simulink model "cruise_control_sim"  (R2017b)
settings: Solver=ode1  StartTime=0.0  StopTime=50  FixedStep=0.1  RelTol=1e-3
values from neighbouring files (symbols this model uses):
  EngineRPM = [1000 1500 2000 2500 3000 3500 4000 4500 5000 5500 6000 6500 ... (13 elements, 1x13)]    [alpha147gta.mat]    (also in cruise_control_external.mat; cruise_control_sim.mat)
  EngineTRQ = [200 220 242 258 260 261 268 285 300 296 290 250 ... (13 elements, 1x13)]    [alpha147gta.mat]    (also in cruise_control_external.mat; cruise_control_sim.mat)
  FinalRatio = 3.733    [alpha147gta.mat]    (also in cruise_control_external.mat; cruise_control_sim.mat)
  GearRatio = [3.5 2.235 1.52 1.156 0.971 0.818]    [alpha147gta.mat]    (also in cruise_control_external.mat; cruise_control_sim.mat)
  Kdrag = 0.4238432    [alpha147gta.mat]    (also in cruise_control_external.mat; cruise_control_sim.mat)
  Ki = 1    [cruise_control.mat]    (also in cruise_control_external.mat = 0.002; cruise_control_sim.mat = 0.002)
  Kp = 1    [cruise_control.mat]    (also in cruise_control_external.mat = 0.4; cruise_control_sim.mat = 0.4)
  Mass = 1360    [alpha147gta.mat]    (also in cruise_control_external.mat; cruise_control_sim.mat)
  WheelRadius = 0.2992    [alpha147gta.mat]    (also in cruise_control_external.mat; cruise_control_sim.mat)
undefined symbols (not defined in the file or in its folder): sigbuilder_block
settings Model: Creator=Rehaan M. Bhimani  LastModifiedBy=Rehaan M. Bhimani

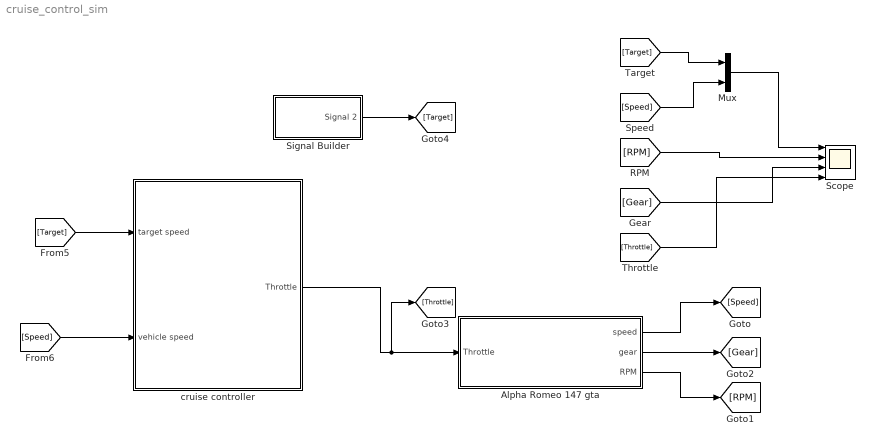
== system cruise_control_sim ==
  Alpha Romeo 147 gta : Subsystem
  Mux : Mux  Inputs=2
  Scope : Scope  NumInputPorts=4
  Signal Builder : Subsystem  Tag=STV Subsys  LoadFcn=sigbuilder_block('load');  StartFcn=sigbuilder_block('start');  StopFcn=sigbuilder_block('stop');  ClipboardFcn=sigbuilder_block('clipboard');  mask(Sigbuilder block){tuvar=[0:10]}
      mask help: Simulink:masks:SigbuilderBlock_MD
      mask init:
      | if ~strcmp(get_param(bdroot(gcbh),'SimulationStatus'),'stopped') tuvar = sigbuilder_block('maskInit'); end
      settings: CopyFcn=sigbuilder_block('copy');  DeleteFcn=sigbuilder_block('delete');  ModelCloseFcn=sigbuilder_block('modelClose');  PreSaveFcn=sigbuilder_block('preSave');  PauseFcn=sigbuilder_block('pause');  ContinueFcn=sigbuilder_block('continue');  NameChangeFcn=sigbuilder_block('namechange');  OpenFcn=sigbuilder_block('open',[404 117.5 550.5 362.5 ]);  CloseFcn=sigbuilder_block('close');
      mask Display: plot(0, 0, 100, 100,[2, 2, 32, 32, 2], [68, 8, 8, 68, 68],[32, 2], [38, 38], [32, 19, 2],[53, 60, 44], [32, 17, 17, 2],[16, 16, 31, 31]);txt = getActiveGroup(gcbh);text(2, 100, txt,'verticalAlignment', 'top');
  "cruise controller " : Subsystem
  wires:
  "cruise controller "/1("Throttle ") -> [Throttle], Alpha Romeo 147 gta/1(Throttle)
  [Target] -> "cruise controller "/1(target speed)
  Alpha Romeo 147 gta/1(speed) -> [Speed]
  Alpha Romeo 147 gta/2(gear) -> [Gear]
  Alpha Romeo 147 gta/3(RPM) -> [RPM]
  [Speed] -> "cruise controller "/2(vehicle speed)
  [Target] -> Mux/1
  [Speed] -> Mux/2
  Mux/1 -> Scope/1
  [RPM] -> Scope/2
  [Gear] -> Scope/3
  [Throttle] -> Scope/4
  Signal Builder/1(Signal 2) -> [Target]

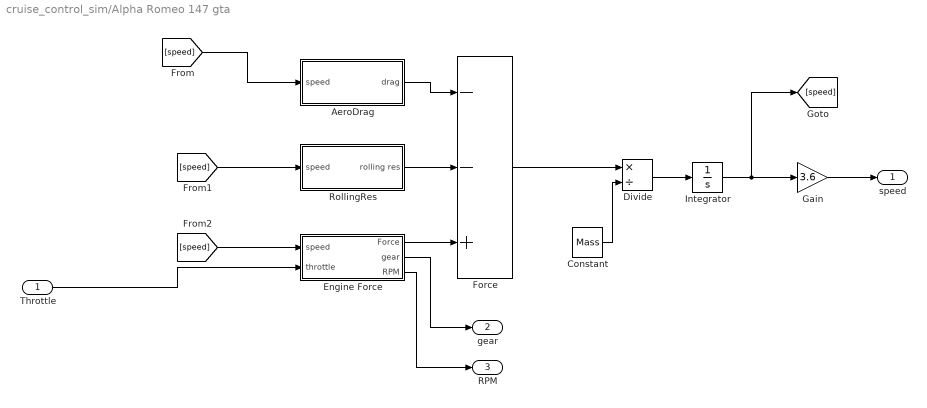
== system cruise_control_sim/Alpha Romeo 147 gta ==
  Throttle : Inport
  AeroDrag : Subsystem
  Constant : Constant  Value=Mass
  Divide : Product  Inputs=*/
  Engine Force : Subsystem
  Force : Sum  Inputs=--+
  Gain : Gain  Gain=3.6
  Integrator : Integrator
  RollingRes : Subsystem
  speed : Outport
  gear : Outport  Port=2
  RPM : Outport  Port=3
  wires:
  Throttle/1 -> Engine Force/2(throttle)
  [speed] -> Engine Force/1(speed)
  Gain/1 -> speed/1
  Force/1 -> Divide/1
  RollingRes/1(rolling res) -> Force/2
  AeroDrag/1(drag) -> Force/1
  [speed] -> RollingRes/1(speed)
  Engine Force/1(Force) -> Force/3
  Divide/1 -> Integrator/1
  Integrator/1 -> [speed], Gain/1
  Constant/1 -> Divide/2
  [speed] -> AeroDrag/1(speed)
  Engine Force/2(gear) -> gear/1
  Engine Force/3(RPM) -> RPM/1

== system cruise_control_sim/Signal Builder ==
  Demux : Demux  Tag=STV Demux  Outputs=1
  FromWs : FromWorkspace  Tag=STV FromWs  VariableName=tuvar  SampleTime=0
      SigBuilderData=|
      | common.afterFinalStr = 'Extrapolate'
      | common.sampleTime = 0
      | dataSet.timeRange = [0 50]
      | dataSet.name = 'Group 1'
      | sbobj.Groups.Name = 'Group 1'
      | sbobj.Groups.Signals.Name = 'Signal 2'
      | sbobj.Groups.Signals.XData = [0 5 5 10 10 20 20 30 30 40 40 50]
      | sbobj.Groups.Signals.YData = [30 30 50 50 80 80 100 100 120 120 140 140]
      | sbobj.Groups.TimeRange = [0 50]
  Signal 2 : Outport  Tag=STV Outport
  wires:
  FromWs/1 -> Demux/1
  Demux/1 -> Signal 2/1

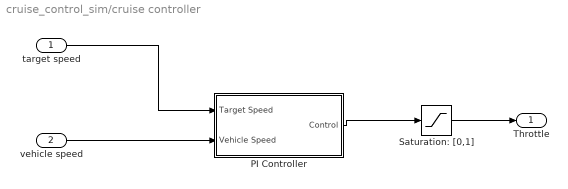
== system cruise_control_sim/cruise controller  ==
  target speed : Inport
  vehicle speed : Inport  Port=2
  PI Controller : Subsystem
  Saturation: [0,1] : Saturate  UpperLimit=1  LowerLimit=0
  "Throttle " : Outport
  wires:
  Saturation: [0,1]/1 -> "Throttle "/1
  target speed/1 -> PI Controller/1(Target Speed)
  vehicle speed/1 -> PI Controller/2(Vehicle Speed)
  PI Controller/1(Control) -> Saturation: [0,1]/1

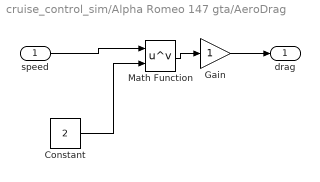
== system cruise_control_sim/Alpha Romeo 147 gta/AeroDrag ==
  speed : Inport
  Constant : Constant  Value=2
  Gain : Gain
  Math Function : Math  Operator=pow  SaturateOnIntegerOverflow=on
  drag : Outport
  wires:
  Gain/1 -> drag/1
  Math Function/1 -> Gain/1
  Constant/1 -> Math Function/2
  speed/1 -> Math Function/1

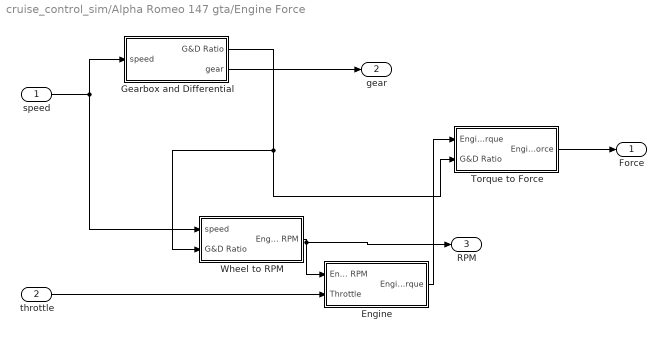
== system cruise_control_sim/Alpha Romeo 147 gta/Engine Force ==
  speed : Inport
  throttle : Inport  Port=2
  Engine : Subsystem
  Gearbox and Differential : Subsystem
  Torque to Force : Subsystem
  Wheel to RPM : Subsystem
  Force : Outport
  gear : Outport  Port=2
  RPM : Outport  Port=3
  wires:
  speed/1 -> Wheel to RPM/1(speed), Gearbox and Differential/1(speed)
  throttle/1 -> Engine/2(Throttle)
  Gearbox and Differential/1(G&D Ratio) -> Torque to Force/2(G&D Ratio), Wheel to RPM/2(G&D Ratio)
  Wheel to RPM/1(Engine RPM) -> RPM/1, Engine/1("Engine RPM ")
  Engine/1(Engine Torque) -> Torque to Force/1(Engine Torque)
  Torque to Force/1(Engine Force) -> Force/1
  Gearbox and Differential/2(gear) -> gear/1

== system cruise_control_sim/Alpha Romeo 147 gta/RollingRes ==
  speed : Inport
  Gain : Gain  Gain=30 * Kdrag
  rolling res : Outport
  wires:
  speed/1 -> Gain/1
  Gain/1 -> rolling res/1

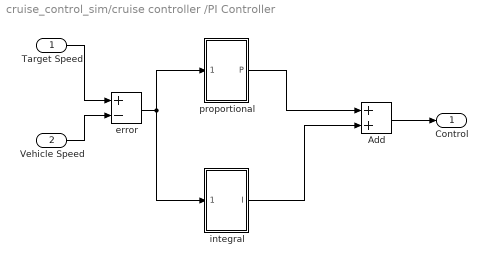
== system cruise_control_sim/cruise controller /PI Controller ==
  Target Speed : Inport
  Vehicle Speed : Inport  Port=2
  Add : Sum
  error : Sum  Inputs=+-
  integral : Subsystem
  proportional : Subsystem
  Control : Outport
  wires:
  Add/1 -> Control/1
  Vehicle Speed/1 -> error/2
  integral/1(I) -> Add/2
  Target Speed/1 -> error/1
  error/1 -> integral/1(error), proportional/1(error)
  proportional/1("P ") -> Add/1

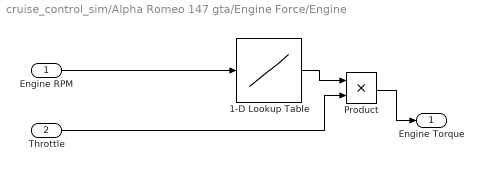
== system cruise_control_sim/Alpha Romeo 147 gta/Engine Force/Engine ==
  "Engine RPM " : Inport
  Throttle : Inport  Port=2
  1-D Lookup Table : Lookup_n-D  NumberOfTableDimensions=1  BreakpointsForDimension1=EngineRPM  Table=EngineTRQ  InterpMethod=Cubic spline  InternalRulePriority=Speed  RndMeth=Simplest  InputSameDT=on
  Product : Product
  Engine Torque : Outport
  wires:
  "Engine RPM "/1 -> 1-D Lookup Table/1
  1-D Lookup Table/1 -> Product/1
  Throttle/1 -> Product/2
  Product/1 -> Engine Torque/1

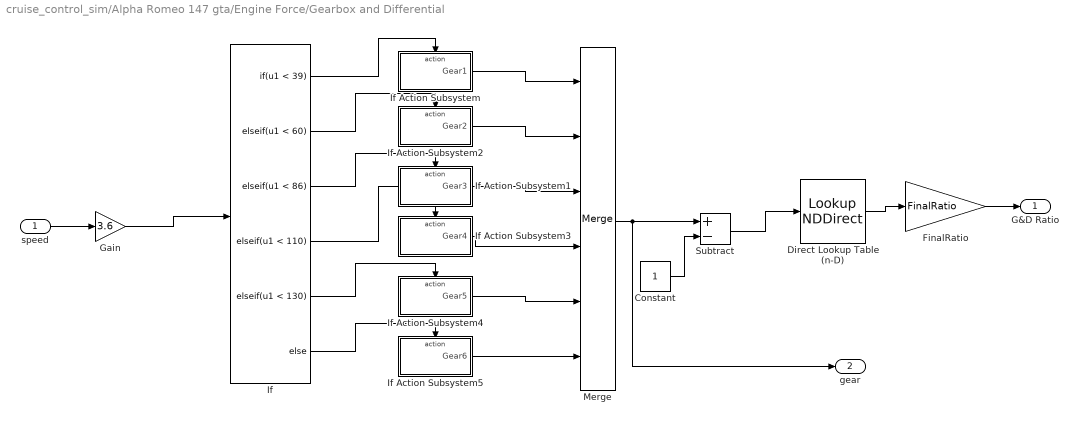
== system cruise_control_sim/Alpha Romeo 147 gta/Engine Force/Gearbox and Differential ==
  speed : Inport
  Constant : Constant
  Direct Lookup Table (n-D) : LookupNDDirect  NumberOfTableDimensions=1  Table=GearRatio
  FinalRatio : Gain  Gain=FinalRatio
  Gain : Gain  Gain=3.6
  If : If  IfExpression=u1 < 39  ElseIfExpressions=u1 < 60, u1 < 86, u1 < 110, u1 < 130
  If Action Subsystem : Subsystem  TreatAsAtomicUnit=on
  If Action Subsystem1 : Subsystem  TreatAsAtomicUnit=on
  If Action Subsystem2 : Subsystem  TreatAsAtomicUnit=on
  If Action Subsystem3 : Subsystem  TreatAsAtomicUnit=on
  If Action Subsystem4 : Subsystem  TreatAsAtomicUnit=on
  If Action Subsystem5 : Subsystem  TreatAsAtomicUnit=on
  Merge : Merge  Inputs=6
  Subtract : Sum  Inputs=+-
  G&D Ratio : Outport
  gear : Outport  Port=2
  wires:
  speed/1 -> Gain/1
  Gain/1 -> If/1
  If/1 -> If Action Subsystem/Action
  If/2 -> If Action Subsystem2/Action
  If/3 -> If Action Subsystem1/Action
  If/4 -> If Action Subsystem3/Action
  If/5 -> If Action Subsystem4/Action
  If/6 -> If Action Subsystem5/Action
  If Action Subsystem/1(Gear1) -> Merge/1
  If Action Subsystem2/1(Gear2) -> Merge/2
  If Action Subsystem1/1("Gear3 ") -> Merge/3
  If Action Subsystem3/1(Gear4) -> Merge/4
  If Action Subsystem4/1(Gear5) -> Merge/5
  If Action Subsystem5/1(Gear6) -> Merge/6
  Merge/1 -> gear/1, Subtract/1
  Constant/1 -> Subtract/2
  Subtract/1 -> Direct Lookup Table (n-D)/1
  Direct Lookup Table (n-D)/1 -> FinalRatio/1
  FinalRatio/1 -> G&D Ratio/1

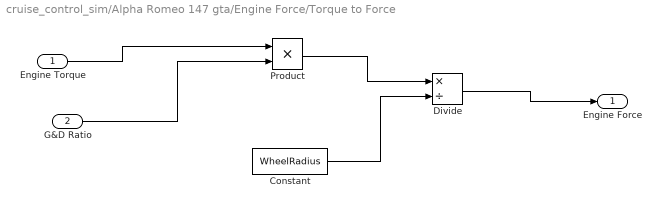
== system cruise_control_sim/Alpha Romeo 147 gta/Engine Force/Torque to Force ==
  Engine Torque : Inport
  G&D Ratio : Inport  Port=2
  Constant : Constant  Value=WheelRadius
  Divide : Product  Inputs=*/
  Product : Product
  Engine Force : Outport
  wires:
  Constant/1 -> Divide/2
  G&D Ratio/1 -> Product/2
  Engine Torque/1 -> Product/1
  Product/1 -> Divide/1
  Divide/1 -> Engine Force/1

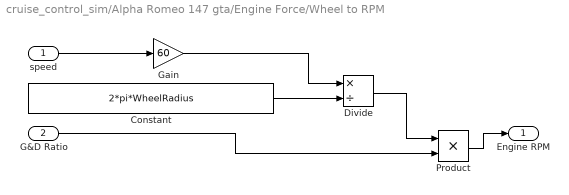
== system cruise_control_sim/Alpha Romeo 147 gta/Engine Force/Wheel to RPM ==
  speed : Inport
  G&D Ratio : Inport  Port=2
  Constant : Constant  Value=2*pi*WheelRadius
  Divide : Product  Inputs=*/
  Gain : Gain  Gain=60
  Product : Product
  Engine RPM : Outport
  wires:
  speed/1 -> Gain/1
  Gain/1 -> Divide/1
  Constant/1 -> Divide/2
  Divide/1 -> Product/1
  G&D Ratio/1 -> Product/2
  Product/1 -> Engine RPM/1

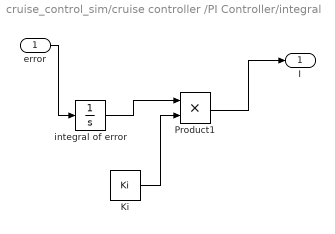
== system cruise_control_sim/cruise controller /PI Controller/integral ==
  error : Inport
  Ki : Constant  Value=Ki
  Product1 : Product
  integral of error : Integrator
  I : Outport
  wires:
  integral of error/1 -> Product1/1
  Ki/1 -> Product1/2
  error/1 -> integral of error/1
  Product1/1 -> I/1

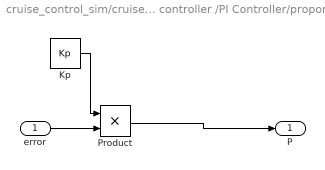
== system cruise_control_sim/cruise controller /PI Controller/proportional ==
  error : Inport
  "Kp " : Constant  Value=Kp
  Product : Product
  "P " : Outport
  wires:
  Product/1 -> "P "/1
  error/1 -> Product/2
  "Kp "/1 -> Product/1

== system cruise_control_sim/Alpha Romeo 147 gta/Engine Force/Gearbox and Differential/If Action Subsystem ==
  Action Port : ActionPort  ActionType=then
  Constant : Constant
  Gear1 : Outport
  wires:
  Constant/1 -> Gear1/1

== system cruise_control_sim/Alpha Romeo 147 gta/Engine Force/Gearbox and Differential/If Action Subsystem1 ==
  Action Port : ActionPort  ActionType=elseif
  Constant : Constant  Value=3
  "Gear3 " : Outport
  wires:
  Constant/1 -> "Gear3 "/1

== system cruise_control_sim/Alpha Romeo 147 gta/Engine Force/Gearbox and Differential/If Action Subsystem2 ==
  Action Port : ActionPort  ActionType=elseif
  Constant : Constant  Value=2
  Gear2 : Outport
  wires:
  Constant/1 -> Gear2/1

== system cruise_control_sim/Alpha Romeo 147 gta/Engine Force/Gearbox and Differential/If Action Subsystem3 ==
  Action Port : ActionPort  ActionType=elseif
  Constant : Constant  Value=4
  Gear4 : Outport
  wires:
  Constant/1 -> Gear4/1

== system cruise_control_sim/Alpha Romeo 147 gta/Engine Force/Gearbox and Differential/If Action Subsystem4 ==
  Action Port : ActionPort  ActionType=elseif
  Constant : Constant  Value=5
  Gear5 : Outport
  wires:
  Constant/1 -> Gear5/1

== system cruise_control_sim/Alpha Romeo 147 gta/Engine Force/Gearbox and Differential/If Action Subsystem5 ==
  Action Port : ActionPort  ActionType=else
  Constant : Constant  Value=6
  Gear6 : Outport
  wires:
  Constant/1 -> Gear6/1
